simulink model "aquaculture_system"  (R2023b)
settings: Solver=VariableStepAuto  StartTime=0.0  StopTime=8640  RelTol=1e-3
values from neighbouring files (symbols this model uses):
  aeration_efficiency = 0.9*0.005    (= 0.0045)    [init.m]
  alpha = 0.015    [init.m]
  biofilter_alkalinity = 0.02    [init.m]
  biofilter_demand = 0.02    [init.m]
  biomass = 3000    [init.m]
  cooling_rate = (cool_water_flow/tank_volume)*rate_of_change_per_degree*1000    (= 0.00898283261803)    [init.m]
  delta_t = 10    [init.m]
  fish_co2_excretion = 1.375*fish_oxygen_consumption    (= 6.20323676681e-06)    [init.m]
  fish_oxygen_consumption = 630.7/(tank_volume*biomass)    (= 4.51144492132e-06)    [init.m]
  metabolic_heat = 5e-7    (= 5e-07)    [init.m]
  ox_kd = 0.01    [init.m]
  ox_ki = 0.02    [init.m]
  ox_kp = 2    [init.m]
  oxygen_0 = 2.0    (= 2)    [init.m]
  oxygen_reference = 5.5    [init.m]
  ph_0 = 7.4    [init.m]
  ph_increase = 0.01    [init.m]
  T_0 = 21.5    [init.m]
  T_ext = 18    [init.m]
  T_in = 14    [init.m]
undefined symbols (not defined in the file or in its folder): DiscIntNeverNeededParam
libraries: slpidlib x1
settings Model: Creator=paco  LastModifiedBy=paco

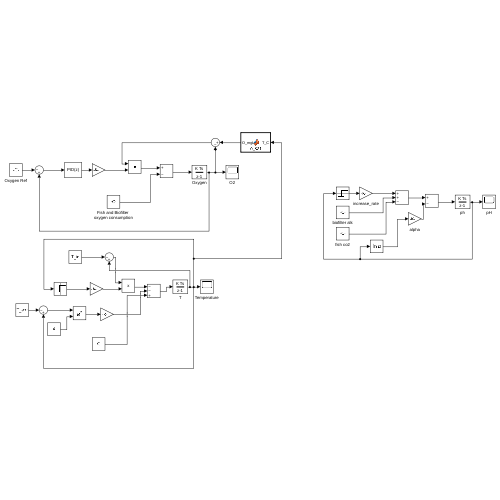
[thumbnail: Simulink's stored preview of the top-level diagram]
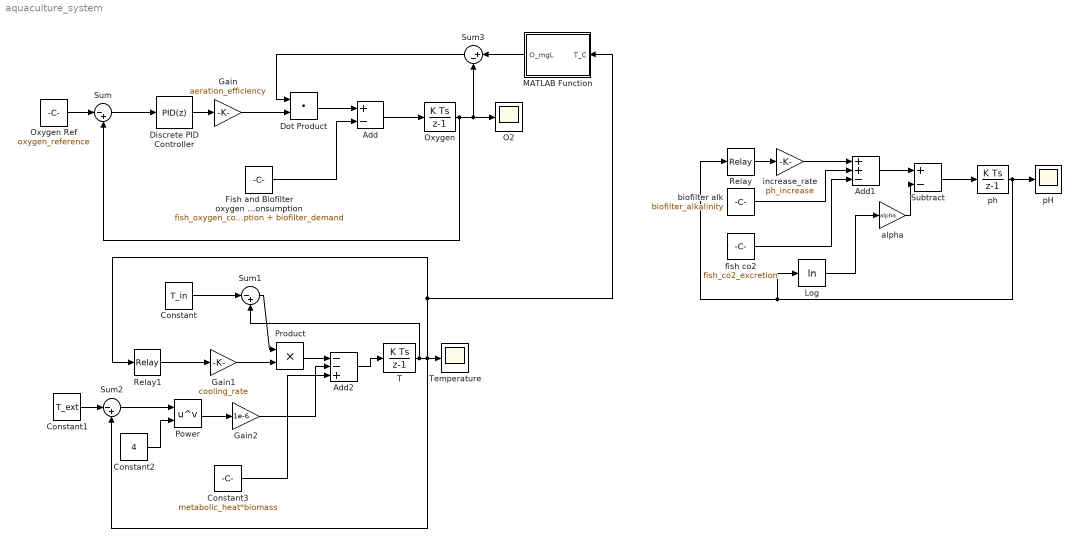
== system aquaculture_system ==
  Add : Sum  Inputs=+-
  Add1 : Sum  Inputs=++-
  Add2 : Sum  Inputs=--+
  Constant : Constant  Value=T_in
  Constant1 : Constant  Value=T_ext
  Constant2 : Constant  Value=4
  Constant3 : Constant  Value=metabolic_heat*biomass
  Discrete PID Controller : slpidlib/PID Controller  Controller=PID  Form=Parallel  TimeDomain=Discrete-time  UseExternalTs=off  SampleTime=delta_t  IntegratorMethod=Forward Euler  FilterMethod=Forward Euler  ControllerParametersSource=internal  P=ox_kp  I=ox_ki  UseKiTs=off  D=ox_kd  N=100  UseFilter=off  TunerSelectOption=Transfer Function Based (PID Tuner App)  InitialConditionSource=internal  InitialConditionForIntegrator=0  InitialConditionForFilter=0  DifferentiatorICPrevScaledInput=0  ExternalReset=none  TrackingMode=off  Kt=1  LimitOutput=off  SatLimitsSource=internal  UpperSaturationLimit=inf  LowerSaturationLimit=-inf  LinearizeAsGain=off  AntiWindupMode=none  Kb=1  LimitIntegrator=off  UpperIntegratorSaturationLimit=inf  LowerIntegratorSaturationLimit=-inf  POutMin=[]  POutMax=[]  IOutMin=[]  IOutMax=[]  DOutMin=[]  DOutMax=[]  NOutMin=[]  NOutMax=[]  SumOutMin=[]  SumOutMax=[]  SaturationOutMin=[]  SaturationOutMax=[]  PParamMin=[]  PParamMax=[]  IParamMin=[]  IParamMax=[]  DParamMin=[]  DParamMax=[]  NParamMin=[]  NParamMax=[]  KbParamMin=[]  KbParamMax=[]  KtParamMin=[]  KtParamMax=[]  KbOutMin=[]  KbOutMax=[]  KtOutMin=[]  KtOutMax=[]  IntegratorOutMin=[]  IntegratorOutMax=[]  FilterOutMin=[]  FilterOutMax=[]  SumI1OutMin=[]  SumI1OutMax=[]  SumI2OutMin=[]  SumI2OutMax=[]  SumI3OutMin=[]  SumI3OutMax=[]  SumI4OutMin=[]  SumI4OutMax=[]  SumDOutMin=[]  SumDOutMax=[]  DifferentiatorOutMin=[]  DifferentiatorOutMax=[]  FilterDiffOutCoefMin=[]  FilterDiffOutCoefMax=[]  ReciprocalOutMin=[]  ReciprocalOutMax=[]  SumDenOutMin=[]  SumDenOutMax=[]  SumNumOutMin=[]  SumNumOutMax=[]  DivideOutMin=[]  DivideOutMax=[]  UdiffTsProdOutMin=[]  UdiffTsProdOutMax=[]  NTsProdOutMin=[]  NTsProdOutMax=[]  UintegralTsProdOutMin=[]  UintegralTsProdOutMax=[]  UngainTsProdOutMin=[]  UngainTsProdOutMax=[]  ClampingZeroOutDataTypeStr=Inherit: Inherit via back propagation  ClampingZeroOutMin=[]  ClampingZeroOutMax=[]  FilterDenConstantOutDataTypeStr=Inherit: Inherit via back propagation  FilterDenConstantOutMin=[]  FilterDenConstantOutMax=[]  PCopyOutDataTypeStr=Inherit: Inherit via back propagation  PCopyOutMin=[]  PCopyOutMax=[]  NCopyOutDataTypeStr=Inherit: Inherit via back propagation  NCopyOutMin=[]  NCopyOutMax=[]  IntegratorContinuousStateAttributes=''  IntegratorStateMustResolveToSignalObject=off  IntegratorRTWStateStorageClass=Auto  FilterContinuousStateAttributes=''  FilterStateMustResolveToSignalObject=off  FilterRTWStateStorageClass=Auto  ParallelPVariant=InternalParameters  IdealPVariant=Disabled  IVariant=InternalParameters  DVariant=InternalParameters  IntegratorVariant=Discrete  SatVariant=Disabled  AWVariant=Passthrough  PCopyVariant=Disabled  TRVariant=Disabled  FdbkBlocksVariant=Forward  IdealPFdbkVariant=Disabled  SatFdbkVariant=Disabled  DerivativeFilterVariant=Differentiator  NVariant=Passthrough  NCopyVariant=Disabled_SignalSpec  FilterICVariant=InternalICsDifferentiator  IntegratorICVariant=InternalICs  ExternalResetVariant=Disabled  TRSumVariant=Passthrough  SumFdbkVariant=Disabled  SumVariant=Sum_PID  TsampFilterVariant=InternalTs  TsampNgainVariant=Passthrough  TsampIntegralVariant=Disabled_SignalSpec  ExternalSaturationOutDataTypeStr=Inherit: Same as second input
      settings: LibrarySourceBlock=simulink/Discrete/Discrete PID Controller
  Dot Product : DotProduct  OutDataTypeStr=Inherit: Inherit via internal rule
  Fish and Biofilter oxygen consumption : Constant  Value=fish_oxygen_consumption + biofilter_demand
  Gain : Gain  Gain=aeration_efficiency
  Gain1 : Gain  Gain=cooling_rate
  Gain2 : Gain  Gain=1e-6
  Log : Math  Operator=log
  MATLAB Function : MATLAB Function  TreatAsAtomicUnit=on
  O2 : Scope
  Oxygen : DiscreteIntegrator  InitialCondition=oxygen_0  SampleTime=delta_t  StateName=Oxygen [mg/L]  ICPrevOutput=DiscIntNeverNeededParam  ICPrevScaledInput=DiscIntNeverNeededParam
  Oxygen Ref : Constant  Value=oxygen_reference
  Power : Math  Operator=pow
  Product : Product
  Relay : Relay  OnSwitchValue=7.2  OffSwitchValue=6.8  OnOutputValue=0  OffOutputValue=1
  Relay1 : Relay  OnSwitchValue=22  OffSwitchValue=21
  Subtract : Sum  Inputs=+-
  Sum : Sum  Inputs=|-+
  Sum1 : Sum  Inputs=|-+
  Sum2 : Sum  Inputs=|-+
  Sum3 : Sum  Inputs=|+-
  T : DiscreteIntegrator  InitialCondition=T_0  SampleTime=delta_t  StateName=Temperature  ICPrevOutput=DiscIntNeverNeededParam  ICPrevScaledInput=DiscIntNeverNeededParam
  Temperature : Scope
  alpha : Gain  Gain=alpha
  biofilter alk : Constant  Value=biofilter_alkalinity
  fish co2 : Constant  Value=fish_co2_excretion
  increase_rate : Gain  Gain=ph_increase
  pH : Scope
  ph : DiscreteIntegrator  InitialCondition=ph_0  SampleTime=delta_t  StateName=ph  ICPrevOutput=DiscIntNeverNeededParam  ICPrevScaledInput=DiscIntNeverNeededParam
  wires:
  Oxygen Ref/1 -> Sum/1
  Sum/1 -> Discrete PID Controller/1
  Discrete PID Controller/1 -> Gain/1
  Fish and Biofilter oxygen consumption/1 -> Add/2
  Add/1 -> Oxygen/1
  Oxygen/1 -> O2/1, Sum3/2, Sum/2
  ph/1 -> Log/1, Relay/1, pH/1
  Relay/1 -> increase_rate/1
  increase_rate/1 -> Add1/1
  biofilter alk/1 -> Add1/2
  fish co2/1 -> Add1/3
  Add1/1 -> Subtract/1
  alpha/1 -> Subtract/2
  Subtract/1 -> ph/1
  Log/1 -> alpha/1
  T/1 -> Sum1/2, Sum2/2, MATLAB Function/1(T_C), Relay1/1, Temperature/1
  Constant/1 -> Sum1/1
  Sum1/1 -> Product/1
  Gain1/1 -> Product/2
  Relay1/1 -> Gain1/1
  Product/1 -> Add2/1
  Constant1/1 -> Sum2/1
  Sum2/1 -> Power/1
  Constant2/1 -> Power/2
  Power/1 -> Gain2/1
  Gain2/1 -> Add2/2
  Constant3/1 -> Add2/3
  Add2/1 -> T/1
  MATLAB Function/1(O_mgL) -> Sum3/1
  Gain/1 -> Dot Product/2
  Dot Product/1 -> Add/1
  Sum3/1 -> Dot Product/1

== matlab function aquaculture_system/MATLAB Function ==
  data: T_C input; O_mgL output
function O_mgL = o_sat(T_C)
    T_K = max(T_C + 273.15, 274); 
    A1 = -173.4292;
    A2 = 249.6339;
    A3 = 143.3483;
    A4 = -21.8492;

    ln_O = A1 + A2 * (100 ./ T_K) + A3 * log(T_K / 100) + A4 * (T_K / 100).^2;
    O_molkg = exp(ln_O);  % mol/kg·atm
    O_mgL = O_molkg * 32 * 1000;  % convert to mg/L
end
